simulink model "rst_sans_ss"  (R2018b)
settings: Solver=VariableStepAuto  StartTime=0.0  StopTime=20  RelTol=1e-3
values from neighbouring files (symbols this model uses):
  A = [0 0 1; 0 -alpha1 0; 0 sig1 -alpha2]    [synthese.m]
  Ad = sysbod.A    [synthese.m]
  alpha2 = 100    [synthese.m]
  B = [0; sig0; 0]    [synthese.m]
  Bd = sysbod.B    [synthese.m]
  C = [1 0 0]    [synthese.m]
  Cd = sysbod.C    [synthese.m]
  Dd = sysbod.D    [synthese.m]
  Fobs = Fe(1:3)    [synthese.m]
  Fobsd = Fed(1:3)    [synthese.m]
  Hobs = -Fe(4)    [synthese.m]
  Hobsd = -Fed(4)    [synthese.m]
  L = acker(A', C',P)'    [synthese.m]
  Ld = acker(Ad', Cd', Pd)'    [synthese.m]
  r0 = x(3)    [aide_resolution_eq_bezout.m]
  r1 = x(4)    [aide_resolution_eq_bezout.m]
  r2 = x(5)    [aide_resolution_eq_bezout.m]
  sp1 = x(2)    [aide_resolution_eq_bezout.m]
  Te = 0.3    [aide_resolution_eq_bezout.m]    (also in synthese.m)
undefined symbols (not defined in the file or in its folder): DiscIntNeverNeededParam
settings Model: Creator=poteaum  LastModifiedBy=poteaum

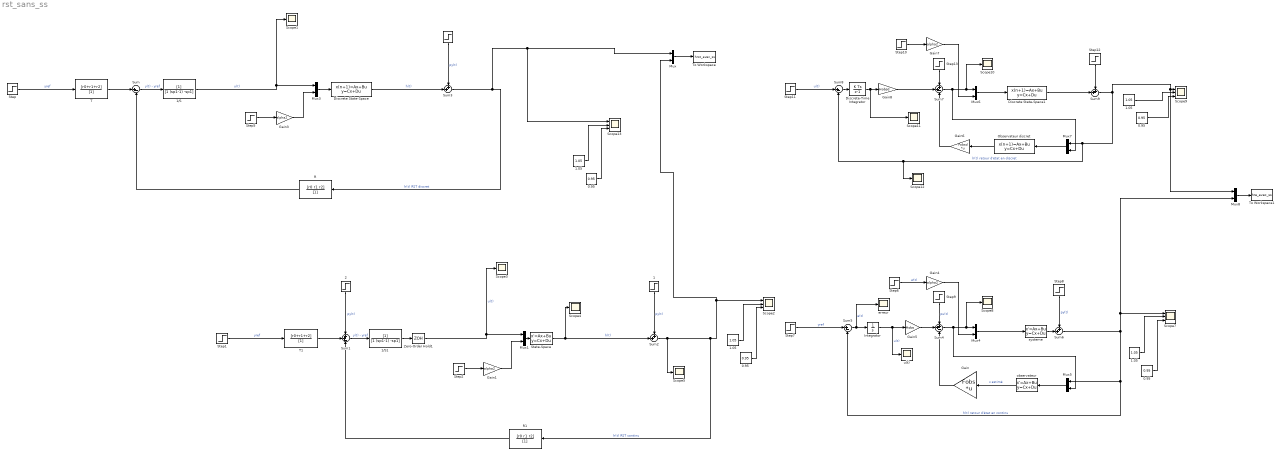
== system rst_sans_ss ==
  " " : Step  Time=0  After=0.1  SampleTime=0
  " 1" : Step  Time=0  After=0.1  SampleTime=0
  " 2" : Step  Time=0  After=0.1  SampleTime=0
  0.95 : Constant  Value=0.95
  "0.95 " : Constant  Value=0.95
  "0.95 " : Constant  Value=0.95
  "0.95 " : Constant  Value=0.95
  1.05 : Constant  Value=1.05
  "1.05 " : Constant  Value=1.05
  "1.05 " : Constant  Value=1.05
  "1.05  " : Constant  Value=1.05
  1/S : DiscreteFilter  Denominator=[1 (sp1-1) -sp1]
  1/S1 : DiscreteFilter  Denominator=[1 (sp1-1) -sp1]
  Discrete State-Space : DiscreteStateSpace  A=Ad  B=Bd  C=Cd  D=Dd  SampleTime=Te
  Discrete State-Space1 : DiscreteStateSpace  A=Ad  B=Bd  C=Cd  D=Dd  SampleTime=Te
  Discrete-Time Integrator : DiscreteIntegrator  SampleTime=Te  ICPrevOutput=DiscIntNeverNeededParam  ICPrevScaledInput=DiscIntNeverNeededParam
  Gain : Gain  Gain=Fobs  Multiplication=Matrix(K*u)
  Gain{1,3..4,7} (4 alike) : Gain  Gain=alpha2
  Gain5 : Gain  Gain=Hobs
  Gain6 : Gain  Gain=Fobsd  Multiplication=Matrix(K*u)
  Gain8 : Gain  Gain=Hobsd
  Integrator : Integrator
  Mux{,1,3..8} (8 alike) : Mux  Inputs=2
  Observateur discret : DiscreteStateSpace  A=Ad-Ld*Cd  B=[Ld Bd(:,1)]  C=eye(3)  D=zeros(3,2)  SampleTime=Te
  R : DiscreteFilter  Numerator=[r0 r1 r2]  Denominator=[1]  SampleTime=Te
  R1 : DiscreteFilter  Numerator=[r0 r1 r2]  Denominator=[1]  SampleTime=Te
  Scope{1,3..5,8,10..12} (8 alike) : Scope
  Scope{2,7,9,13} (4 alike) : Scope  NumInputPorts=3
  State-Space : StateSpace  A=A  B=[B E]  C=C  D=zeros(1,2)  InitialCondition=0
  Step : Step  Time=0  SampleTime=0
  Step1 : Step  Time=0  SampleTime=0
  Step10 : Step  Time=0  After=0.01  SampleTime=Te
  Step11 : Step  Time=0  SampleTime=Te
  Step12 : Step  Time=10  After=0.1  SampleTime=0
  Step13 : Step  Time=0  After=0.1  SampleTime=0
  Step2 : Step  Time=0  After=0.01  SampleTime=0
  Step5 : Step  Time=0  After=0.01  SampleTime=0
  Step6 : Step  Time=0  After=0.01  SampleTime=0
  Step7 : Step  Time=0  SampleTime=0
  Step8 : Step  Time=10  After=0.1  SampleTime=Te
  Step9 : Step  Time=0  After=0.1  SampleTime=Te
  Sum : Sum  Inputs=|+-
  Sum1 : Sum  Inputs=++-
  Sum{2..3,6,9} (4 alike) : Sum  Inputs=++|
  Sum4 : Sum  Inputs=++-
  Sum5 : Sum  Inputs=|+-
  Sum7 : Sum  Inputs=++-
  Sum8 : Sum  Inputs=|+-
  T : DiscreteFilter  Numerator=[r0+r1+r2]  Denominator=[1]  SampleTime=Te
  T1 : DiscreteFilter  Numerator=[r0+r1+r2]  Denominator=[1]  SampleTime=Te
  To Workspace : ToWorkspace  VariableName=hrst_avec_ss  SaveFormat=Structure With Time  SampleTime=Te
  To Workspace1 : ToWorkspace  VariableName=hre_avec_ss  SaveFormat=Structure With Time  SampleTime=-1
  Zero-Order Hold1 : ZeroOrderHold  SampleTime=-1
  erreur : Scope
  observateur : StateSpace  A=A-L*C  B=[L B]  C=eye(3)  D=zeros(3,2)  InitialCondition=[0.1;0.1;0.1]  AbsoluteTolerance=1
  systeme : StateSpace  A=A  B=[B E]  C=C  D=zeros(1,2)  InitialCondition=[0;0;0]
  u(t) : Scope
  wires:
  R/1 -> Sum/2
  1/S/1 -> Mux3/1, Scope1/1  "u(t)"
  Sum3/1 -> R/1, Scope13/1, Mux/1  "h(t) RST discret"
  Sum/1 -> 1/S/1  "y(t) - yref"
  T/1 -> Sum/1
  " "/1 -> Sum3/1  "py(t)"
  Step/1 -> T/1  "yref"
  Discrete State-Space/1 -> Sum3/2  "h(t)"
  Step1/1 -> T1/1  "yref"
  Sum1/1 -> 1/S1/1  "y(t) - yref"
  " 1"/1 -> Sum2/1  "py(t)"
  1/S1/1 -> Zero-Order Hold1/1
  R1/1 -> Sum1/3
  Zero-Order Hold1/1 -> Mux1/1, Scope3/1  "u(t)"
  State-Space/1 -> Sum2/2, Scope4/1  "h(t)"
  Sum2/1 -> Scope5/1, R1/1, Scope2/1, Mux/2  "h(t) RST continu"
  T1/1 -> Sum1/2
  Mux/1 -> To Workspace/1
  Mux1/1 -> State-Space/1
  Step2/1 -> Gain1/1
  Gain1/1 -> Mux1/2
  Step5/1 -> Gain3/1
  Gain3/1 -> Mux3/2
  Mux3/1 -> Discrete State-Space/1
  Step6/1 -> Gain4/1  "w(t)"
  Gain4/1 -> Mux4/2
  Mux4/1 -> systeme/1
  observateur/1 -> Gain/1  "x estimé"
  Sum4/1 -> Mux5/2, Scope8/1, Mux4/1
  Gain/1 -> Sum4/3
  Mux5/1 -> observateur/1
  Step7/1 -> Sum5/1  "yref"
  Sum5/1 -> erreur/1, Integrator/1  "e(t)"
  Integrator/1 -> u(t)/1, Gain5/1  "u(t)"
  Sum6/1 -> Sum5/2, Mux5/1, Mux8/2, Scope7/1  "h(t) retour d'état en continu"
  systeme/1 -> Sum6/2
  Step8/1 -> Sum6/1  "py(t)"
  Step9/1 -> Sum4/1  "pu(t)"
  " 2"/1 -> Sum1/1  "py(t)"
  Step10/1 -> Gain7/1
  Gain7/1 -> Mux6/2
  Sum7/1 -> Mux7/2, Scope10/1, Mux6/1
  Gain6/1 -> Sum7/3
  Sum9/1 -> Scope12/1, Sum8/2, Mux7/1, Mux8/1, Scope9/1  "h(t) retour d'état en discret"
  Step11/1 -> Sum8/1  "u(t)"
  Step13/1 -> Sum7/1
  Discrete State-Space1/1 -> Sum9/2
  Discrete-Time Integrator/1 -> Scope11/1, Gain8/1
  Observateur discret/1 -> Gain6/1
  Mux6/1 -> Discrete State-Space1/1
  Step12/1 -> Sum9/1
  Mux7/1 -> Observateur discret/1
  Sum8/1 -> Discrete-Time Integrator/1
  Gain8/1 -> Sum7/2
  Gain5/1 -> Sum4/2
  "1.05 "/1 -> Scope9/2
  0.95/1 -> Scope9/3
  1.05/1 -> Scope7/2
  "0.95 "/1 -> Scope7/3
  "0.95 "/1 -> Scope2/3
  "1.05  "/1 -> Scope2/2
  "0.95 "/1 -> Scope13/3
  "1.05 "/1 -> Scope13/2
  Mux8/1 -> To Workspace1/1
